simulink model "ejemplo2"  (R2025b)
settings: Solver=VariableStepAuto  StartTime=0.0  StopTime=20.0  RelTol=1e-3
settings DataIOCC: ExternalInput=[ut]  LoadExternalInput=on  SaveFormat=Array  SaveState=on

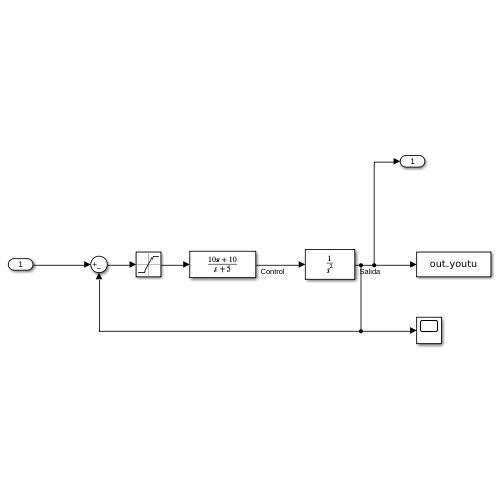
[thumbnail: Simulink's stored preview of the top-level diagram]
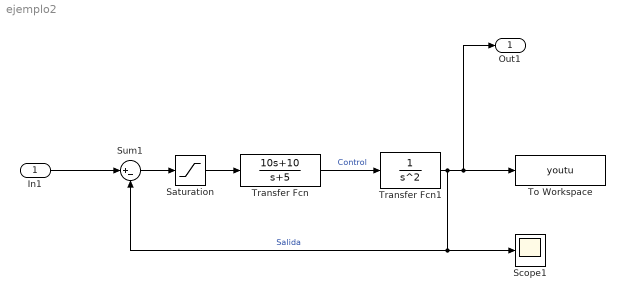
== system ejemplo2 ==
  In1 : Inport  OutMin=[-1]  OutMax=[7.5]
  Saturation : Saturate  UpperLimit=1  LowerLimit=-1
  Scope1 : Scope
      settings: ActiveDisplayYMinimum=-121.71323975326436  ActiveDisplayYMaximum=252.79490980068149
  Sum1 : Sum  Inputs=|+-
  To Workspace : ToWorkspace  VariableName=youtu  SampleTime=-1
  Transfer Fcn : TransferFcn  Numerator=[10 10]  Denominator=[1 5]
  Transfer Fcn1 : TransferFcn  Denominator=[1 0 0]
  Out1 : Outport
  wires:
  Transfer Fcn/1 -> Transfer Fcn1/1  "Control"
  Transfer Fcn1/1 -> To Workspace/1, Out1/1, Scope1/1, Sum1/2  "Salida"
  Saturation/1 -> Transfer Fcn/1
  Sum1/1 -> Saturation/1
  In1/1 -> Sum1/1
